simulink model "ESP_RTW"  (Simulink 10.1)
settings: Solver=ode1  StartTime=0.0  StopTime=inf  FixedStep=0.001  RelTol=1e-3
PreLoadFcn:
  | vehicle = 'Car'; if ~length(which('cmcmd')), cmenv; end
  | ESP_RTW_bus
  | ESP_RTW_params
InitFcn:
  | vehicle = 'Car'; if ~length(which('cmcmd')), cmenv; end
  | ESP_RTW_bus
  | ESP_RTW_params
values from neighbouring files (symbols this model uses):
  Area_Front = 23    [ESP_RTW_params.m]
  Area_Rear = 23    [ESP_RTW_params.m]
  ay_max_off = 4.0    (= 4)    [ESP_RTW_params.m]
  ay_max_on = 4.8    [ESP_RTW_params.m]
  ay_per_mu_max_off = 6    [ESP_RTW_params.m]
  ay_per_mu_max_on = 7    [ESP_RTW_params.m]
  Brake_ratio = 0.7    [ESP_RTW_params.m]
  brake_valve_ctrl_kP = 0.5    [ESP_RTW_params.m]
  cat1mode1_higher = 9    [ESP_RTW_params.m]
  cat1mode1_lower = 8    [ESP_RTW_params.m]
  cat1mode2_higher = 6    [ESP_RTW_params.m]
  cat1mode2_lower = 5    [ESP_RTW_params.m]
  cat1mode3_higher = 4    [ESP_RTW_params.m]
  cat1mode3_lower = 3    [ESP_RTW_params.m]
  cat2mode1_higher = 6    [ESP_RTW_params.m]
  cat2mode1_lower = 5.5    [ESP_RTW_params.m]
  cat2mode2_higher = 3    [ESP_RTW_params.m]
  cat2mode2_lower = 2.5    [ESP_RTW_params.m]
  cat2mode3_higher = 1    [ESP_RTW_params.m]
  cat2mode3_lower = 0.5    [ESP_RTW_params.m]
  delta_vel = 10    [ESP_RTW_params.m]
  diff_lock_fac = 1000    [ESP_RTW_params.m]
  diff_lock_off = 3    [ESP_RTW_params.m]
  diff_lock_on = 4    [ESP_RTW_params.m]
  ESP_ctrl_kD = 0    [ESP_RTW_params.m]
  ESP_ctrl_kI = -0.0001    [ESP_RTW_params.m]
  ESP_ctrl_kP = 0.4    [ESP_RTW_params.m]
  ESP_ctrl_restore_kI = 0.6    [ESP_RTW_params.m]
  ESP_min_throttle_fac = 0    [ESP_RTW_params.m]
  f_ax = 0.003    [ESP_RTW_params.m]
  f_slip = 1    [ESP_RTW_params.m]
  g = 9.81    [ESP_RTW_params.m]
  higherlimit_highvel = 2    [ESP_RTW_params.m]
  higherlimit_lowvel = 7    [ESP_RTW_params.m]
  highervel_fac = 0.04    [ESP_RTW_params.m]
  highervelocity_fac = 1.04    [ESP_RTW_params.m]
  limit_acc = 2    [ESP_RTW_params.m]
  limit_selectlow = 38    [ESP_RTW_params.m]
  limit_starting = 10    [ESP_RTW_params.m]
  limit_vdiff = 1    [ESP_RTW_params.m]
  locktime_throttle = 2    [ESP_RTW_params.m]
  lowerlimit_highvel = 1    [ESP_RTW_params.m]
  lowerlimit_lowvel = 6    [ESP_RTW_params.m]
  lowervel_fac = 0.02    [ESP_RTW_params.m]
  lowervelocity_fac = 1.02    [ESP_RTW_params.m]
  min_throttle = 0.05    [ESP_RTW_params.m]
  MPS2KMPH = 3.6    [ESP_RTW_params.m]
  MSR_ctrl_kD = 0    [ESP_RTW_params.m]
  MSR_ctrl_kI = 0    [ESP_RTW_params.m]
  MSR_ctrl_kP = 0.1    [ESP_RTW_params.m]
  MSR_min_throttle_fac = 0.2    [ESP_RTW_params.m]
  PID_kD_sideslip = 0    [ESP_RTW_params.m]
  PID_kD_yawrate = 0    [ESP_RTW_params.m]
  PID_kI_sideslip = 0    [ESP_RTW_params.m]
  PID_kI_yawrate = 0    [ESP_RTW_params.m]
  PID_kP_sideslip = 2550*0.55    (= 1402.5)    [ESP_RTW_params.m]
  PID_kP_yawrate = 6650*0.275    (= 1828.75)    [ESP_RTW_params.m]
  RADpS2RpM = 60/(2*pi)    (= 9.54929658551)    [ESP_RTW_params.m]
  rBrake = 0.1    [ESP_RTW_params.m]
  RpM2RADpS = (2*pi)/60    (= 0.10471975512)    [ESP_RTW_params.m]
  SH_SL_switch = 15    [ESP_RTW_params.m]
  sideslip_vel_corr = 5/6    (= 0.833333333333)    [ESP_RTW_params.m]
  sidesplip_deviation_max = 3    [ESP_RTW_params.m]
  sku_HA = 0.08   +offset    (= 0.08)    [ESP_RTW_params.m]
  sku_off_HA = 0.04   +offset    (= 0.04)    [ESP_RTW_params.m]
  sku_off_VA = 0.03   +offset    (= 0.03)    [ESP_RTW_params.m]
  sku_VA = 0.10   +offset    (= 0.1)    [ESP_RTW_params.m]
  SteerAng_Out = [-0.6 -0.6 -0.5 -0.41 -0.34 -0.27 -0.2 -0.13 -0.06 0 0.06 0.13 0.2 0.27 0.34 0.41 0.5 0.6 0.6]    [ESP_RTW_params.m]
  SteerWheelAng_In = [-15 -8 -7 -6 -5 -4 -3 -2 -1 0 1 2 3 4 5 6 7 8 15]    [ESP_RTW_params.m]
  t_Sensor = triggertime    (= 0.001)    [ESP_RTW_params.m]
  threshold_carpitch_off = 0.05    [ESP_RTW_params.m]
  threshold_carpitch_on = 0.1    [ESP_RTW_params.m]
  threshold_deceleration = -1    [ESP_RTW_params.m]
  threshold_eng_trq_off = 25    [ESP_RTW_params.m]
  threshold_eng_trq_on = 30    [ESP_RTW_params.m]
  threshold_velocity_off = -0.01    [ESP_RTW_params.m]
  threshold_velocity_on = 0.01    [ESP_RTW_params.m]
  v_min = 5    [ESP_RTW_params.m]
  Valve_LUTin_HA = [0 sku_off_HA-1e-5 ,sku_off_HA, sku_HA, sku_HA+1e-5, sko_HA-1e-5, sko_HA , sko_open_HA]    [ESP_RTW_params.m]
  Valve_LUTin_VA = [0 sku_off_VA-1e-5 ,sku_off_VA, sku_VA, sku_VA+1e-5, sko_VA-1e-5, sko_VA , sko_open_VA]    [ESP_RTW_params.m]
  ValveIn_abbau = 1    [ESP_RTW_params.m]
  ValveIn_aufbau_long = 0    [ESP_RTW_params.m]
  ValveIn_aufbau_short = 0.85    [ESP_RTW_params.m]
  ValveIn_LUTout_HA = [0, 0,   0.2,    0.6,    1.0,    1.0,     1.0,    1.0]    [ESP_RTW_params.m]
  ValveIn_LUTout_VA = [0, 0,   0.2,    0.4,    1.0,    1.0,     1.0,    1.0]    [ESP_RTW_params.m]
  ValveOut_abbau = 1    [ESP_RTW_params.m]
  ValveOut_aufbau_long = 0    [ESP_RTW_params.m]
  ValveOut_aufbau_short = 0.85    [ESP_RTW_params.m]
  ValveOut_LUTout_HA = [0, 0,   0,      0,      0,     0,      0.3,    1.0]    [ESP_RTW_params.m]
  ValveOut_LUTout_VA = [0, 0,   0,      0,      0,     0,      0.3,    1.0]    [ESP_RTW_params.m]
  vel_char_lim_high = 150    [ESP_RTW_params.m]
  vel_char_lim_low = 25    [ESP_RTW_params.m]
  wheelspeed_filter_denom = [1 1]    [ESP_RTW_params.m]
  wheelspeed_filter_num = [ones(1,20)/20]    [ESP_RTW_params.m]
  yawrate_deviation_max = 1    [ESP_RTW_params.m]
  yawrate_vel_corr = 0.5    [ESP_RTW_params.m]
undefined symbols (not defined in the file or in its folder): InitialConditionForIntegrator
libraries: CarMaker4SL x133, simulink x47, simulink_extras x6
(part 2 of 4)

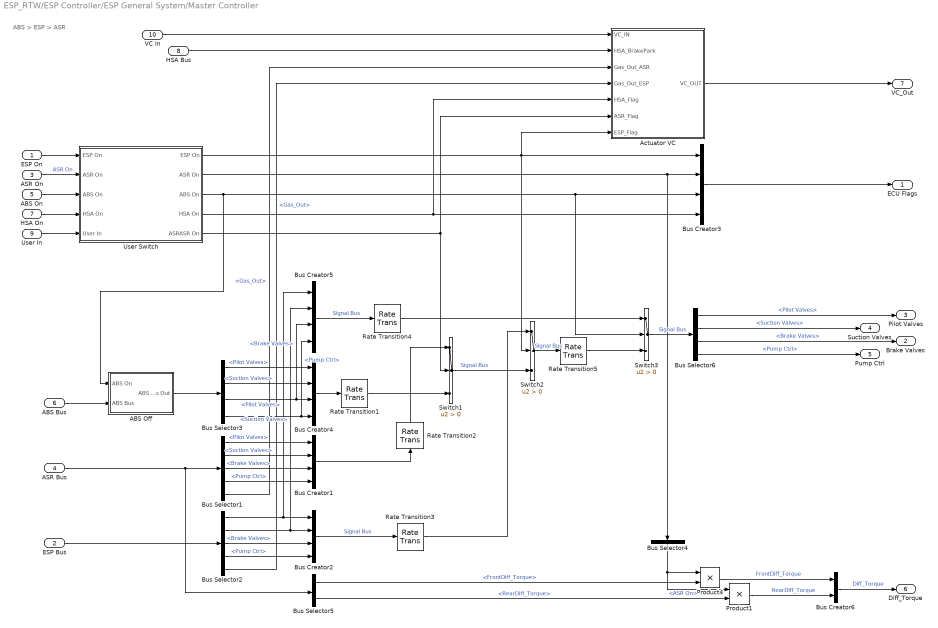
== system ESP_RTW/ESP Controller/ESP General System/Master Controller ==
  note: ABS > ESP > ASR
  ESP On : Inport
  ESP Bus : Inport  Port=2
  ASR On : Inport  Port=3
  ASR Bus : Inport  Port=4
  ABS On : Inport  Port=5
  ABS Bus : Inport  Port=6
  HSA On : Inport  Port=7
  HSA Bus : Inport  Port=8
  User In : Inport  Port=9
  VC In : Inport  Port=10
  ABS Off : Subsystem
  Actuator VC : Subsystem
  Bus Creator{1..5} (5 alike) : BusCreator  Inputs=4
  Bus Creator6 : BusCreator  Inputs=2
  Bus Selector1 : BusSelector  OutputSignals=Pilot Valves,Suction Valves,Brake Valves,Pump Ctrl,Gas_Out
  Bus Selector2 : BusSelector  OutputSignals=Pilot Valves,Suction Valves,Brake Valves,Pump Ctrl,Gas_Out
  Bus Selector3 : BusSelector  OutputSignals=Pilot Valves,Suction Valves,Brake Valves,Pump Ctrl
  Bus Selector4 : BusSelector  OutputSignals=ASR On
  Bus Selector5 : BusSelector  OutputSignals=Diff_Torque.FrontDiff_Torque,Diff_Torque.RearDiff_Torque
  Bus Selector6 : BusSelector  OutputSignals=Pilot Valves,Suction Valves,Brake Valves,Pump Ctrl
  Product1 : Product  RndMeth=Zero
  Product4 : Product  RndMeth=Zero
  Rate Transition{1..5} (5 alike) : RateTransition
  Switch1 : Switch  Criteria=u2 > Threshold
  Switch2 : Switch  Criteria=u2 > Threshold
  Switch3 : Switch  Criteria=u2 > Threshold
  User Switch : Subsystem
  ECU Flags : Outport  VectorParamsAs1DForOutWhenUnconnected=off
  Brake Valves : Outport  Port=2  VectorParamsAs1DForOutWhenUnconnected=off
  Pilot Valves : Outport  Port=3  VectorParamsAs1DForOutWhenUnconnected=off
  Suction Valves : Outport  Port=4  VectorParamsAs1DForOutWhenUnconnected=off
  Pump Ctrl : Outport  Port=5  VectorParamsAs1DForOutWhenUnconnected=off
  Diff_Torque : Outport  Port=6  VectorParamsAs1DForOutWhenUnconnected=off
  VC_Out : Outport  Port=7  VectorParamsAs1DForOutWhenUnconnected=off
  wires:
  Rate Transition5/1 -> Switch3/3
  Rate Transition4/1 -> Switch3/1
  Rate Transition3/1 -> Switch2/1
  ABS Off/1(ABS Bus Out) -> Bus Selector3/1
  Bus Selector4/1 -> Product4/1, Product1/1  "<ASR On>"
  Bus Creator6/1 -> Diff_Torque/1  "Diff_Torque"
  Product1/1 -> Bus Creator6/2  "RearDiff_Torque"
  Product4/1 -> Bus Creator6/1  "FrontDiff_Torque"
  Bus Selector5/2 -> Product1/2  "<RearDiff_Torque>"
  Bus Selector5/1 -> Product4/2  "<FrontDiff_Torque>"
  User Switch/4("HSA On ") -> Actuator VC/5(HSA_Flag), Bus Creator3/4
  HSA On/1 -> User Switch/4(HSA On)
  HSA Bus/1 -> Actuator VC/2(HSA_BrakePark)
  User Switch/2("ASR On ") -> Bus Selector4/1, Bus Creator3/2
  User In/1 -> User Switch/5(User In)
  ABS On/1 -> User Switch/3(ABS On)
  ASR On/1 -> User Switch/2(ASR On)  "ASR On"
  ESP On/1 -> User Switch/1(ESP On)
  User Switch/1("ESP On ") -> Switch2/2, Bus Creator3/1, Actuator VC/7(ESP_Flag)
  User Switch/5(ASRASR On) -> Switch1/2, Actuator VC/6(ASR_Flag)
  User Switch/3("ABS On ") -> Switch3/2, Bus Creator3/3, ABS Off/1(ABS On)
  Bus Selector2/5 -> Actuator VC/4(Gas_Out_ESP)  "<Gas_Out>"
  Bus Selector1/5 -> Actuator VC/3(Gas_Out_ASR)  "<Gas_Out>"
  Switch3/1 -> Bus Selector6/1  "Signal Bus"
  Rate Transition1/1 -> Switch1/3
  Rate Transition2/1 -> Switch1/1
  Bus Creator4/1 -> Rate Transition1/1
  Bus Creator1/1 -> Rate Transition2/1
  Bus Creator5/1 -> Rate Transition4/1  "Signal Bus"
  Switch2/1 -> Rate Transition5/1  "Signal Bus"
  Bus Selector1/4 -> Bus Creator1/4  "<Pump Ctrl>"
  Bus Selector1/3 -> Bus Creator1/3  "<Brake Valves>"
  Bus Selector1/2 -> Bus Creator1/2  "<Suction Valves>"
  Bus Selector1/1 -> Bus Creator1/1  "<Pilot Valves>"
  ASR Bus/1 -> Bus Selector1/1, Bus Selector5/1
  Bus Creator2/1 -> Rate Transition3/1  "Signal Bus"
  Switch1/1 -> Switch2/3  "Signal Bus"
  Bus Selector3/2 -> Bus Creator4/2  "<Suction Valves>"
  Bus Selector3/1 -> Bus Creator4/1  "<Pilot Valves>"
  ABS Bus/1 -> ABS Off/2(ABS Bus)
  Bus Selector3/4 -> Bus Creator4/4, Bus Creator5/4  "<Pump Ctrl>"
  Bus Selector3/3 -> Bus Creator4/3, Bus Creator5/3  "<Brake Valves>"
  Bus Selector6/4 -> Pump Ctrl/1  "<Pump Ctrl>"
  Bus Selector6/3 -> Brake Valves/1  "<Brake Valves>"
  Bus Selector6/2 -> Suction Valves/1  "<Suction Valves>"
  Bus Selector6/1 -> Pilot Valves/1  "<Pilot Valves>"
  Bus Selector2/4 -> Bus Creator2/4  "<Pump Ctrl>"
  Bus Selector2/3 -> Bus Creator2/3  "<Brake Valves>"
  Bus Selector2/2 -> Bus Creator2/2, Bus Creator5/2  "<Suction Valves>"
  Bus Selector2/1 -> Bus Creator2/1, Bus Creator5/1  "<Pilot Valves>"
  ESP Bus/1 -> Bus Selector2/1
  VC In/1 -> Actuator VC/1(VC_IN)
  Actuator VC/1(VC_OUT) -> VC_Out/1
  Bus Creator3/1 -> ECU Flags/1

== system ESP_RTW/ESP Controller/ESP General System/Signal Handling ==
  ESP In : Inport
  Vehicle Params : Inport  Port=2
  " " : simulink_extras/Transformations/Degrees to Radians
  "  " : simulink_extras/Transformations/Degrees to Radians
  "   " : Gain  Gain=RpM2RADpS
  "     " : Gain  Gain=RpM2RADpS
  "      " : Gain  Gain=RpM2RADpS
  Bus Creator : BusCreator  Inputs=4
  Bus Creator1 : BusCreator  Inputs=4
  Bus Creator2 : BusCreator  Inputs=6
  Bus Creator3 : BusCreator  Inputs=2
  Bus Creator4 : BusCreator  Inputs=2
  Bus Creator5 : BusCreator  Inputs=1
  Bus Selector1 : BusSelector  OutputSignals=WheelSpd FL [rpm],WheelSpd FR [rpm],WheelSpd RL [rpm],WheelSpd RR [rpm],Master Cylinder Pressure [bar],Throttle Valve Position [%],Sensor Longitudinal acceleration [g],Engine Speed [rpm],GearState [-],Torque Converter Speed [rpm],Sensor YawRate [degs],Steering Wheel Angle [deg],Sensor Lateral acceleration [g],Cylinder Pressure FL [bar],Cylinder Pressure FR [bar],Cylinder Pressure RL [bar],Cylinder Pressure RR [bar],Engine crankshaft output torque [Nm]
  Bus Selector2 : BusSelector  OutputSignals=SteeringGeometry
  Bus Selector3 : BusSelector  OutputSignals=SteerWheelAng_In,SteerAng_Out
  Gain2 : Gain  Gain=g  SaturateOnIntegerOverflow=on  OutDataTypeStr=Inherit: Same as input  ParamDataTypeStr=Inherit: Same as input
  Gain7 : Gain  Gain=g  SaturateOnIntegerOverflow=on  OutDataTypeStr=Inherit: Same as input  ParamDataTypeStr=Inherit: Same as input
  Lookup Table Dynamic : simulink/Lookup Tables/Lookup Table Dynamic  LookUpMeth=Interpolation-Use End Values  OutDataTypeStr=fixdt('double')  OutputDataTypeScalingMode=Specify via dialog  OutDataType=fixdt('double')  OutScaling=2^-10  DoSatur=off
  Termiator : Terminator
  Terminator1 : Terminator
  Terminator2 : Terminator
  Terminator4 : Terminator
  rpmin2rad/s : Gain  Gain=RpM2RADpS
  vquer_VA3 : Gain  Gain=0.01
  Signal Bus ESP : Outport  VectorParamsAs1DForOutWhenUnconnected=off
  Signal Bus ASR : Outport  Port=2  VectorParamsAs1DForOutWhenUnconnected=off
  Signal Bus ABS : Outport  Port=3  VectorParamsAs1DForOutWhenUnconnected=off
  Signal Bus HSA : Outport  Port=4  VectorParamsAs1DForOutWhenUnconnected=off
  wires:
  Bus Selector3/1 -> Lookup Table Dynamic/2  "<SteerWheelAng_In>"
  Bus Selector3/2 -> Lookup Table Dynamic/3  "<SteerAng_Out>"
  Bus Selector2/1 -> Bus Selector3/1  "<SteeringGeometry>"
  Vehicle Params/1 -> Bus Selector2/1
  Bus Creator5/1 -> Signal Bus HSA/1
  Bus Creator4/1 -> Signal Bus ABS/1
  Bus Selector1/18 -> Bus Creator5/1  "<Engine crankshaft output torque [Nm]>"
  Bus Creator3/1 -> Signal Bus ASR/1
  Bus Creator/1 -> Bus Creator3/1, Bus Creator4/1  "WheelSpeeds"
  Bus Creator2/1 -> Signal Bus ESP/1
  Bus Creator1/1 -> Bus Creator2/6  "Wheel Cylinder Pressure"
  Bus Selector1/14 -> Bus Creator1/1  "<Cylinder Pressure FL [bar]>"
  Bus Selector1/16 -> Bus Creator1/3  "<Cylinder Pressure RL [bar]>"
  Bus Selector1/17 -> Bus Creator1/4  "<Cylinder Pressure RR [bar]>"
  Bus Selector1/15 -> Bus Creator1/2  "<Cylinder Pressure FR [bar]>"
  vquer_VA3/1 -> Bus Creator3/2, Bus Creator2/1  "Throttle Position"
  Gain2/1 -> Bus Creator2/4  "ay [m/s^2]"
  " "/1 -> Bus Creator2/2  "Yaw Rate"
  Lookup Table Dynamic/1 -> Bus Creator2/3  "Steer Angle"
  ESP In/1 -> Bus Selector1/1
  Bus Selector1/6 -> vquer_VA3/1  "<Throttle Valve Position [%]>"
  Gain7/1 -> Bus Creator2/5, Bus Creator4/2  "ax [m/s^2]"
  "      "/1 -> Bus Creator/4  "WheelSpd_RR"
  "     "/1 -> Bus Creator/3  "WheelSpd_RL"
  "   "/1 -> Bus Creator/2  "WheelSpd_FR"
  Bus Selector1/13 -> Gain2/1  "<Sensor Lateral acceleration [g]>"
  Bus Selector1/12 -> "  "/1  "<Steering Wheel Angle [deg]>"
  Bus Selector1/11 -> " "/1  "<Sensor YawRate [degs]>"
  Bus Selector1/10 -> Termiator/1  "<Torque Converter Speed [rpm]>"
  Bus Selector1/9 -> Terminator1/1  "<GearState [-]>"
  Bus Selector1/8 -> Terminator2/1  "<Engine Speed [rpm]>"
  Bus Selector1/5 -> Terminator4/1  "<Master Cylinder Pressure [bar]>"
  Bus Selector1/7 -> Gain7/1  "<Sensor Longitudinal acceleration [g]>"
  Bus Selector1/4 -> "      "/1  "<WheelSpd RR [rpm]>"
  Bus Selector1/3 -> "     "/1  "<WheelSpd RL [rpm]>"
  Bus Selector1/2 -> "   "/1  "<WheelSpd FR [rpm]>"
  Bus Selector1/1 -> rpmin2rad/s/1  "<WheelSpd FL [rpm]>"
  rpmin2rad/s/1 -> Bus Creator/1  "WheelSpd_FL"
  "  "/1 -> Lookup Table Dynamic/1

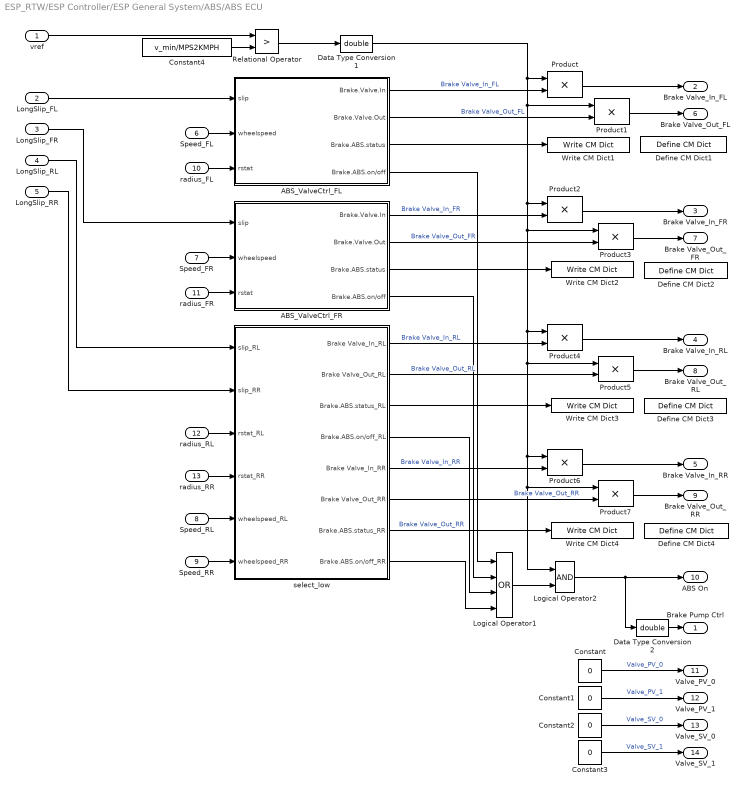
== system ESP_RTW/ESP Controller/ESP General System/ABS/ABS ECU ==
  vref : Inport
  LongSlip_FL : Inport  Port=2
  LongSlip_FR : Inport  Port=3
  LongSlip_RL : Inport  Port=4
  LongSlip_RR : Inport  Port=5
  Speed_FL : Inport  Port=6
  Speed_FR : Inport  Port=7
  Speed_RL : Inport  Port=8
  Speed_RR : Inport  Port=9
  radius_FL : Inport  Port=10
  radius_FR : Inport  Port=11
  radius_RL : Inport  Port=12
  radius_RR : Inport  Port=13
  ABS_ValveCtrl_FL : Subsystem
  ABS_ValveCtrl_FR : Subsystem
  Constant{,1..3} (4 alike) : Constant  Value=0
  Constant4 : Constant  Value=v_min/MPS2KMPH
  Data Type Conversion1 : DataTypeConversion  OutDataTypeStr=double
  Data Type Conversion2 : DataTypeConversion  OutDataTypeStr=double
  Define CM Dict1 : CarMaker4SL/Define CM Dict  xname=ESP.ABS.Status_FL  xmono=off  xtype=Char  xdvaplace=None  xnstates=4  xfirststate=0  xinitial=0
  Define CM Dict2 : CarMaker4SL/Define CM Dict  xname=ESP.ABS.Status_FR  xmono=off  xtype=Char  xdvaplace=None  xnstates=4  xfirststate=0  xinitial=0
  Define CM Dict3 : CarMaker4SL/Define CM Dict  xname=ESP.ABS.Status_RL  xmono=off  xtype=Char  xdvaplace=None  xnstates=4  xfirststate=0  xinitial=0
  Define CM Dict4 : CarMaker4SL/Define CM Dict  xname=ESP.ABS.Status_RR  xmono=off  xtype=Char  xdvaplace=None  xnstates=4  xfirststate=0  xinitial=0
  Logical Operator1 : Logic  Operator=OR  Inputs=4  AllPortsSameDT=off
  Logical Operator2 : Logic  AllPortsSameDT=off
  Product{,1..7} (8 alike) : Product  SaturateOnIntegerOverflow=on  OutDataTypeStr=Inherit: Same as first input
  Relational Operator : RelationalOperator  Operator=>  RndMeth=Nearest
  Write CM Dict1 : CarMaker4SL/Write CM Dict  xname=ESP.ABS.Status_FL  xsync=off
  Write CM Dict2 : CarMaker4SL/Write CM Dict  xname=ESP.ABS.Status_FR  xsync=off
  Write CM Dict3 : CarMaker4SL/Write CM Dict  xname=ESP.ABS.Status_RL  xsync=off
  Write CM Dict4 : CarMaker4SL/Write CM Dict  xname=ESP.ABS.Status_RR  xsync=off
  select_low : Subsystem
  Brake Pump Ctrl : Outport  VectorParamsAs1DForOutWhenUnconnected=off
  Brake Valve_In_FL : Outport  Port=2  VectorParamsAs1DForOutWhenUnconnected=off
  Brake Valve_In_FR : Outport  Port=3  VectorParamsAs1DForOutWhenUnconnected=off
  Brake Valve_In_RL : Outport  Port=4  VectorParamsAs1DForOutWhenUnconnected=off
  Brake Valve_In_RR : Outport  Port=5  VectorParamsAs1DForOutWhenUnconnected=off
  Brake Valve_Out_FL : Outport  Port=6  VectorParamsAs1DForOutWhenUnconnected=off
  Brake Valve_Out_FR : Outport  Port=7  VectorParamsAs1DForOutWhenUnconnected=off
  Brake Valve_Out_RL : Outport  Port=8  VectorParamsAs1DForOutWhenUnconnected=off
  Brake Valve_Out_RR : Outport  Port=9  VectorParamsAs1DForOutWhenUnconnected=off
  ABS On : Outport  Port=10  VectorParamsAs1DForOutWhenUnconnected=off
  Valve_PV_0 : Outport  Port=11  VectorParamsAs1DForOutWhenUnconnected=off
  Valve_PV_1 : Outport  Port=12  VectorParamsAs1DForOutWhenUnconnected=off
  Valve_SV_0 : Outport  Port=13  VectorParamsAs1DForOutWhenUnconnected=off
  Valve_SV_1 : Outport  Port=14  VectorParamsAs1DForOutWhenUnconnected=off
  wires:
  Logical Operator2/1 -> Data Type Conversion2/1, ABS On/1
  Logical Operator1/1 -> Logical Operator2/2
  Constant3/1 -> Valve_SV_1/1  "Valve_SV_1"
  Constant2/1 -> Valve_SV_0/1  "Valve_SV_0"
  Constant1/1 -> Valve_PV_1/1  "Valve_PV_1"
  Constant/1 -> Valve_PV_0/1  "Valve_PV_0"
  vref/1 -> Relational Operator/1
  Speed_RR/1 -> select_low/6(wheelspeed_RR)
  Speed_RL/1 -> select_low/5(wheelspeed_RL)
  radius_RR/1 -> select_low/4(rstat_RR)
  radius_RL/1 -> select_low/3(rstat_RL)
  radius_FR/1 -> ABS_ValveCtrl_FR/3(rstat)
  Speed_FR/1 -> ABS_ValveCtrl_FR/2(wheelspeed)
  radius_FL/1 -> ABS_ValveCtrl_FL/3(rstat)
  Speed_FL/1 -> ABS_ValveCtrl_FL/2(wheelspeed)
  Product2/1 -> Brake Valve_In_FR/1
  Product/1 -> Brake Valve_In_FL/1
  ABS_ValveCtrl_FL/3(Brake.ABS.status) -> Write CM Dict1/1
  LongSlip_RR/1 -> select_low/2(slip_RR)
  LongSlip_RL/1 -> select_low/1(slip_RL)
  LongSlip_FR/1 -> ABS_ValveCtrl_FR/1(slip)
  LongSlip_FL/1 -> ABS_ValveCtrl_FL/1(slip)
  Product1/1 -> Brake Valve_Out_FL/1
  Product3/1 -> Brake Valve_Out_FR/1
  Product4/1 -> Brake Valve_In_RL/1
  Product5/1 -> Brake Valve_Out_RL/1
  Product6/1 -> Brake Valve_In_RR/1
  Product7/1 -> Brake Valve_Out_RR/1
  select_low/6(Brake Valve_Out_RR) -> Product7/2  "Brake Valve_Out_RR"
  select_low/5(Brake Valve_In_RR) -> Product6/2  "Brake Valve_In_RR"
  select_low/2(Brake Valve_Out_RL) -> Product5/2  "Brake Valve_Out_RL"
  select_low/1(Brake Valve_In_RL) -> Product4/2  "Brake Valve_In_RL"
  ABS_ValveCtrl_FR/2(Brake.Valve.Out) -> Product3/2  "Brake Valve_Out_FR"
  ABS_ValveCtrl_FR/1(Brake.Valve.In) -> Product2/2  "Brake Valve_In_FR"
  ABS_ValveCtrl_FL/2(Brake.Valve.Out) -> Product1/2  "Brake Valve_Out_FL"
  ABS_ValveCtrl_FL/1(Brake.Valve.In) -> Product/2  "Brake Valve_In_FL"
  Relational Operator/1 -> Data Type Conversion1/1
  Constant4/1 -> Relational Operator/2
  select_low/8(Brake.ABS.on/off_RR) -> Logical Operator1/4
  select_low/4(Brake.ABS.on/off_RL) -> Logical Operator1/3
  ABS_ValveCtrl_FR/4(Brake.ABS.on/off) -> Logical Operator1/2
  ABS_ValveCtrl_FL/4(Brake.ABS.on/off) -> Logical Operator1/1
  ABS_ValveCtrl_FR/3(Brake.ABS.status) -> Write CM Dict2/1
  select_low/3(Brake.ABS.status_RL) -> Write CM Dict3/1
  select_low/7(Brake.ABS.status_RR) -> Write CM Dict4/1  "Brake Valve_Out_RR"
  Data Type Conversion1/1 -> Product1/1, Product2/1, Product3/1, Product4/1, Product5/1, Logical Operator2/1, Product7/1, Product6/1, Product/1
  Data Type Conversion2/1 -> Brake Pump Ctrl/1

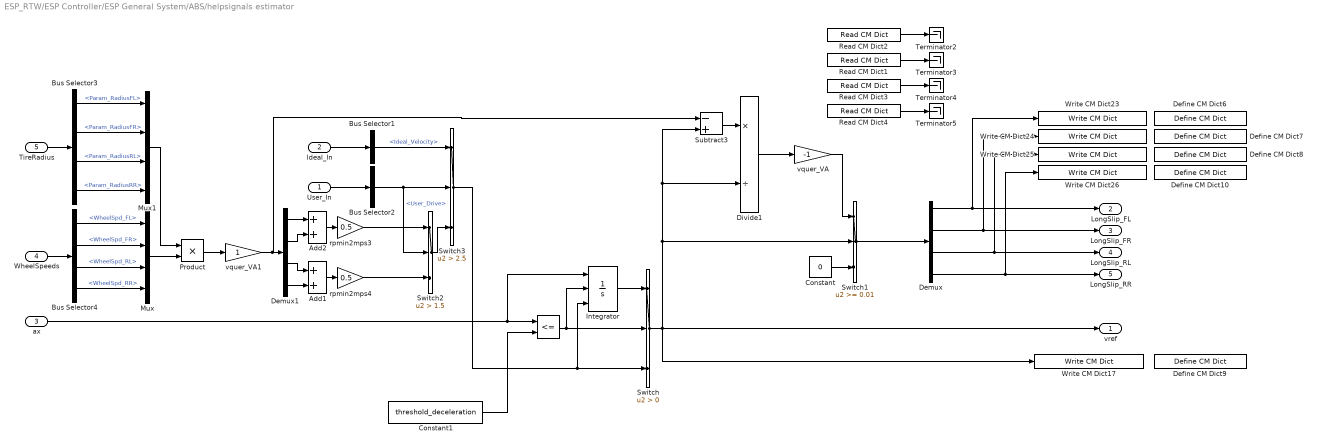
== system ESP_RTW/ESP Controller/ESP General System/ABS/helpsignals estimator ==
  User_In : Inport
  Ideal_In : Inport  Port=2
  ax : Inport  Port=3
  WheelSpeeds : Inport  Port=4
  TireRadius : Inport  Port=5
  " " : RelationalOperator  Operator=<=  OutDataTypeStr=boolean  RndMeth=Nearest
  Add1 : Sum
  Add2 : Sum
  Bus Selector1 : BusSelector  OutputSignals=Ideal_Velocity.Ideal_Velocity
  Bus Selector2 : BusSelector  OutputSignals=User_Drive
  Bus Selector3 : BusSelector  OutputSignals=Param_RadiusFL,Param_RadiusFR,Param_RadiusRL,Param_RadiusRR
  Bus Selector4 : BusSelector  OutputSignals=WheelSpd_FL,WheelSpd_FR,WheelSpd_RL,WheelSpd_RR
  Constant : Constant  Value=0
  Constant1 : Constant  Value=threshold_deceleration
  Define CM Dict10 : CarMaker4SL/Define CM Dict  xname=ESP.ABS.LongSlip_RR  xmono=off  xtype=Double4  xdvaplace=VC  xnstates=0  xfirststate=0  xinitial=0
  Define CM Dict6 : CarMaker4SL/Define CM Dict  xname=ESP.ABS.LongSlip_FL  xmono=off  xtype=Double4  xdvaplace=VC  xnstates=0  xfirststate=0  xinitial=0
  Define CM Dict7 : CarMaker4SL/Define CM Dict  xname=ESP.ABS.LongSlip_FR  xmono=off  xtype=Double4  xdvaplace=VC  xnstates=0  xfirststate=0  xinitial=0
  Define CM Dict8 : CarMaker4SL/Define CM Dict  xname=ESP.ABS.LongSlip_RL  xmono=off  xtype=Double4  xdvaplace=VC  xnstates=0  xfirststate=0  xinitial=0
  Define CM Dict9 : CarMaker4SL/Define CM Dict  xname=ESP.ABS.v_ref  xunit=m/s  xmono=off  xtype=Double4  xdvaplace=VC  xnstates=0  xfirststate=0  xinitial=0
  Demux : Demux
  Demux1 : Demux
  Divide1 : Product  Inputs=*/
  Integrator : Integrator  ExternalReset=rising  InitialConditionSource=external
  Mux : Mux
  Mux1 : Mux
  Product : Product  RndMeth=Zero
  Read CM Dict1 : CarMaker4SL/Read CM Dict  xname=Car.LongSlipFR  xsync=off
  Read CM Dict2 : CarMaker4SL/Read CM Dict  xname=Car.LongSlipFL  xsync=off
  Read CM Dict3 : CarMaker4SL/Read CM Dict  xname=Car.LongSlipRL  xsync=off
  Read CM Dict4 : CarMaker4SL/Read CM Dict  xname=Car.LongSlipRR  xsync=off
  Subtract3 : Sum  Inputs=-+
  Switch : Switch  Criteria=u2 > Threshold
  Switch1 : Switch  Threshold=0.01
  Switch2 : Switch  Criteria=u2 > Threshold  Threshold=1.5
  Switch3 : Switch  Criteria=u2 > Threshold  Threshold=2.5
  Terminator{2..5} (4 alike) : Terminator
  Write CM Dict17 : CarMaker4SL/Write CM Dict  xname=ESP.ABS.v_ref  xsync=off
  Write CM Dict23 : CarMaker4SL/Write CM Dict  xname=ESP.ABS.LongSlip_FL  xsync=off
  Write CM Dict24 : CarMaker4SL/Write CM Dict  xname=ESP.ABS.LongSlip_FR  xsync=off
  Write CM Dict25 : CarMaker4SL/Write CM Dict  xname=ESP.ABS.LongSlip_RL  xsync=off
  Write CM Dict26 : CarMaker4SL/Write CM Dict  xname=ESP.ABS.LongSlip_RR  xsync=off
  rpmin2mps3 : Gain  Gain=0.5
  rpmin2mps4 : Gain  Gain=0.5
  vquer_VA : Gain  Gain=-1
  vquer_VA1 : Gain
  vref : Outport  VectorParamsAs1DForOutWhenUnconnected=off
  LongSlip_FL : Outport  Port=2  VectorParamsAs1DForOutWhenUnconnected=off
  LongSlip_FR : Outport  Port=3  VectorParamsAs1DForOutWhenUnconnected=off
  LongSlip_RL : Outport  Port=4  VectorParamsAs1DForOutWhenUnconnected=off
  LongSlip_RR : Outport  Port=5  VectorParamsAs1DForOutWhenUnconnected=off
  wires:
  Integrator/1 -> Switch/1
  Constant1/1 -> " "/2
  rpmin2mps4/1 -> Switch2/3
  rpmin2mps3/1 -> Switch2/1
  Bus Selector4/1 -> Mux/1  "<WheelSpd_FL>"
  Bus Selector4/2 -> Mux/2  "<WheelSpd_FR>"
  Bus Selector4/3 -> Mux/3  "<WheelSpd_RL>"
  Bus Selector4/4 -> Mux/4  "<WheelSpd_RR>"
  WheelSpeeds/1 -> Bus Selector4/1
  Bus Selector3/1 -> Mux1/1  "<Param_RadiusFL>"
  Bus Selector3/4 -> Mux1/4  "<Param_RadiusRR>"
  Bus Selector3/3 -> Mux1/3  "<Param_RadiusRL>"
  Bus Selector3/2 -> Mux1/2  "<Param_RadiusFR>"
  TireRadius/1 -> Bus Selector3/1
  Ideal_In/1 -> Bus Selector1/1
  Bus Selector1/1 -> Switch3/1  "<Ideal_Velocity>"
  Switch2/1 -> Switch3/3
  Add2/1 -> rpmin2mps3/1
  Bus Selector2/1 -> Switch3/2, Switch2/2  "<User_Drive>"
  Add1/1 -> rpmin2mps4/1
  User_In/1 -> Bus Selector2/1
  Demux1/2 -> Add2/2
  Demux1/1 -> Add2/1
  Read CM Dict4/1 -> Terminator5/1
  Read CM Dict3/1 -> Terminator4/1
  Read CM Dict1/1 -> Terminator3/1
  Read CM Dict2/1 -> Terminator2/1
  " "/1 -> Switch/2, Integrator/2
  vquer_VA1/1 -> Demux1/1, Subtract3/1
  Demux/4 -> Write CM Dict26/1, LongSlip_RR/1
  Demux/3 -> Write CM Dict25/1, LongSlip_RL/1
  Demux/2 -> Write CM Dict24/1, LongSlip_FR/1
  Demux/1 -> Write CM Dict23/1, LongSlip_FL/1
  Constant/1 -> Switch1/3
  Switch1/1 -> Demux/1
  Switch/1 -> Write CM Dict17/1, vref/1, Switch1/2, Divide1/2, Subtract3/2
  Demux1/4 -> Add1/2
  Demux1/3 -> Add1/1
  Switch3/1 -> Switch/3, Integrator/3
  ax/1 -> " "/1, Integrator/1
  vquer_VA/1 -> Switch1/1
  Divide1/1 -> vquer_VA/1
  Subtract3/1 -> Divide1/1
  Mux/1 -> Product/2
  Mux1/1 -> Product/1
  Product/1 -> vquer_VA1/1

== system ESP_RTW/ESP Controller/ESP General System/ASR/BMR ECU ==
  Throttle : Inport
  WheelVelocity [kmph] : Inport  Port=2
  User_In : Inport  Port=3
  Ideal_In : Inport  Port=4
  BMR Controller : Subsystem
  BMR logic : Subsystem
  Bus Creator : BusCreator  Inputs=8
  Bus Creator1 : BusCreator  Inputs=2
  Bus Creator2 : BusCreator  Inputs=2
  Bus Creator3 : BusCreator  Inputs=2
  Differential Lock : Subsystem
  Signal Mapping : Subsystem
  BMR On : Outport  VectorParamsAs1DForOutWhenUnconnected=off
  Brake Valves : Outport  Port=2  VectorParamsAs1DForOutWhenUnconnected=off
  Pilot Valves : Outport  Port=3  VectorParamsAs1DForOutWhenUnconnected=off
  Suctions Valves : Outport  Port=4  VectorParamsAs1DForOutWhenUnconnected=off
  Pump Ctrl : Outport  Port=5  VectorParamsAs1DForOutWhenUnconnected=off
  Diff_Torque : Outport  Port=6  VectorParamsAs1DForOutWhenUnconnected=off
  wires:
  User_In/1 -> Signal Mapping/1(User_In), Differential Lock/1(User_In), BMR Controller/1(User_In)
  BMR logic/2(BMR On) -> BMR On/1, BMR Controller/3(BMR On)
  BMR logic/1(mode) -> BMR Controller/2(mode)
  Throttle/1 -> BMR logic/5(Throttle position)
  Signal Mapping/4(v_UndrivenR) -> BMR logic/4(v_undrivenR)
  Signal Mapping/3(v_UndrivenL) -> BMR logic/3(v_undrivenL)
  Signal Mapping/2(v_DrivenR) -> BMR logic/2(v_drivenR), Differential Lock/3(v_DrivenR)
  Signal Mapping/1(v_DrivenL) -> BMR logic/1(v_drivenL), Differential Lock/2(v_DrivenL)
  Ideal_In/1 -> Signal Mapping/3(Ideal_In)
  Bus Creator3/1 -> Diff_Torque/1
  Differential Lock/2(RearDiff_Torque) -> Bus Creator3/2  "RearDiff_Torque"
  Differential Lock/1(FrontDiff_Torque) -> Bus Creator3/1  "FrontDiff_Torque"
  WheelVelocity [kmph]/1 -> Signal Mapping/2(WheelVelocity)
  Bus Creator1/1 -> Suctions Valves/1
  Bus Creator2/1 -> Pilot Valves/1
  BMR Controller/13(Pump Ctrl) -> Pump Ctrl/1  "PumpCtrl"
  BMR Controller/12(Valve_SV_1) -> Bus Creator1/2  "Valve_SV_1"
  BMR Controller/11(Valve_SV_0) -> Bus Creator1/1  "Valve_SV_0"
  BMR Controller/10(Valve_PV_1) -> Bus Creator2/2  "Valve_PV_1"
  BMR Controller/9(Valve_PV_0) -> Bus Creator2/1  "Valve_PV_0"
  BMR Controller/8(Brake Valve_Out_RR) -> Bus Creator/8  "Valve_Out_RR"
  BMR Controller/7(Brake Valve_Out_RL) -> Bus Creator/7  "Valve_Out_RL"
  BMR Controller/6(Brake Valve_Out_FR) -> Bus Creator/6  "Valve_Out_FR"
  BMR Controller/5(Brake Valve_Out_FL) -> Bus Creator/5  "Valve_Out_FL"
  BMR Controller/4(Brake Valve_In_RR) -> Bus Creator/4  "Valve_In_RR"
  BMR Controller/3(Brake Valve_In_RL) -> Bus Creator/3  "Valve_In_RL"
  BMR Controller/2(Brake Valve_In_FR) -> Bus Creator/2  "Valve_In_FR"
  BMR Controller/1(Brake Valve_In_FL) -> Bus Creator/1  "Valve_In_FL"
  Bus Creator/1 -> Brake Valves/1

== system ESP_RTW/ESP Controller/ESP General System/ASR/MSR ECU ==
  Throttle Position : Inport
  WheelVelocity [kmph] : Inport  Port=2
  User_In : Inport  Port=3
  Ideal_In : Inport  Port=4
  MSR logic : Subsystem
  MSR/Gas Controller : Subsystem
  Signal Mapping : Subsystem
  Gas_out : Outport  VectorParamsAs1DForOutWhenUnconnected=off
  MSR On : Outport  Port=2  VectorParamsAs1DForOutWhenUnconnected=off
  wires:
  MSR logic/3(hold torque) -> MSR/Gas Controller/4(hold Gas)
  MSR logic/2(reduce torque) -> MSR/Gas Controller/3(close Gas)
  MSR logic/1(Pseudo_slip) -> MSR/Gas Controller/2(Pseudo_Slip)
  Signal Mapping/4(v_UndrivenR) -> MSR logic/4(v_undrivenR)
  Signal Mapping/3(v_UndrivenL) -> MSR logic/3(v_undrivenL)
  Signal Mapping/2(v_DrivenR) -> MSR logic/2(v_drivenR)
  Signal Mapping/1(v_DrivenL) -> MSR logic/1(v_drivenL)
  Ideal_In/1 -> Signal Mapping/3(Ideal_In)
  User_In/1 -> Signal Mapping/2(User_In)
  WheelVelocity [kmph]/1 -> Signal Mapping/1(WheelVelocity)
  MSR/Gas Controller/2(Gas_Out) -> Gas_out/1
  MSR/Gas Controller/1(MSR_On) -> MSR On/1
  Throttle Position/1 -> MSR/Gas Controller/1(Throttle_position)

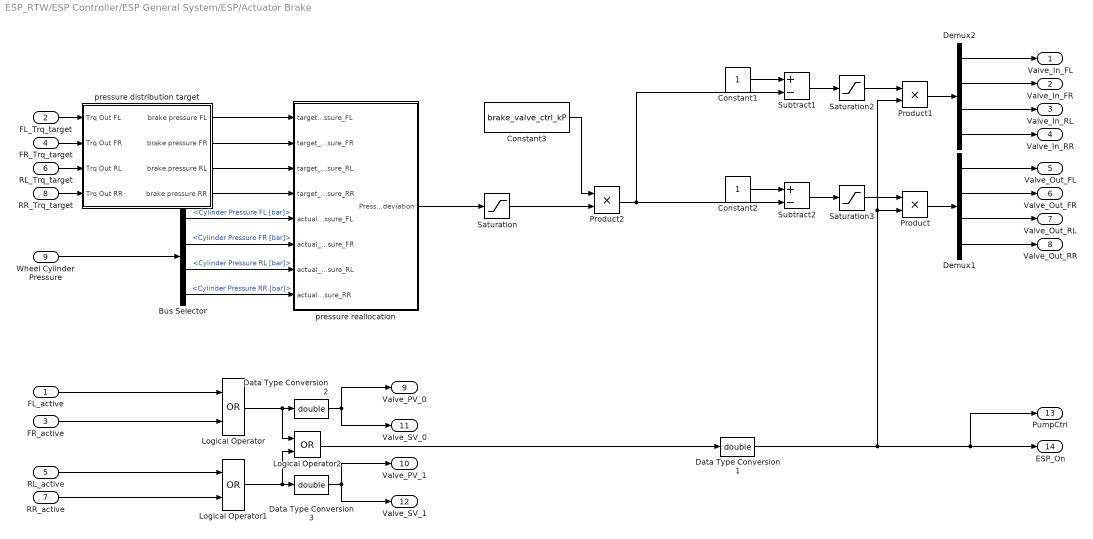
== system ESP_RTW/ESP Controller/ESP General System/ESP/Actuator Brake ==
  FL_active : Inport
  FL_Trq_target : Inport  Port=2
  FR_active : Inport  Port=3
  FR_Trq_target : Inport  Port=4
  RL_active : Inport  Port=5
  RL_Trq_target : Inport  Port=6
  RR_active : Inport  Port=7
  RR_Trq_target : Inport  Port=8
  Wheel Cylinder Pressure : Inport  Port=9
  Bus Selector : BusSelector  OutputSignals=Cylinder Pressure FL [bar],Cylinder Pressure FR [bar],Cylinder Pressure RL [bar],Cylinder Pressure RR [bar]
  Constant1 : Constant
  Constant2 : Constant
  Constant3 : Constant  Value=brake_valve_ctrl_kP
  Data Type Conversion1 : DataTypeConversion  OutDataTypeStr=double
  Data Type Conversion2 : DataTypeConversion  OutDataTypeStr=double
  Data Type Conversion3 : DataTypeConversion  OutDataTypeStr=double
  Demux1 : Demux
  Demux2 : Demux
  Logical Operator : Logic  Operator=OR  AllPortsSameDT=off
  Logical Operator1 : Logic  Operator=OR  AllPortsSameDT=off
  Logical Operator2 : Logic  Operator=OR  AllPortsSameDT=off
  Product : Product  RndMeth=Zero
  Product1 : Product  RndMeth=Zero
  Product2 : Product  RndMeth=Zero
  Saturation : Saturate  UpperLimit=500  LowerLimit=0
  Saturation2 : Saturate  UpperLimit=1  LowerLimit=0
  Saturation3 : Saturate  UpperLimit=1  LowerLimit=0
  Subtract1 : Sum  Inputs=+-
  Subtract2 : Sum  Inputs=+-
  pressure distribution target : Subsystem
  pressure reallocation : Subsystem
  Valve_In_FL : Outport  VectorParamsAs1DForOutWhenUnconnected=off
  Valve_In_FR : Outport  Port=2  VectorParamsAs1DForOutWhenUnconnected=off
  Valve_In_RL : Outport  Port=3  VectorParamsAs1DForOutWhenUnconnected=off
  Valve_In_RR : Outport  Port=4  VectorParamsAs1DForOutWhenUnconnected=off
  Valve_Out_FL : Outport  Port=5  VectorParamsAs1DForOutWhenUnconnected=off
  Valve_Out_FR : Outport  Port=6  VectorParamsAs1DForOutWhenUnconnected=off
  Valve_Out_RL : Outport  Port=7  VectorParamsAs1DForOutWhenUnconnected=off
  Valve_Out_RR : Outport  Port=8  VectorParamsAs1DForOutWhenUnconnected=off
  Valve_PV_0 : Outport  Port=9  VectorParamsAs1DForOutWhenUnconnected=off
  Valve_PV_1 : Outport  Port=10  VectorParamsAs1DForOutWhenUnconnected=off
  Valve_SV_0 : Outport  Port=11  VectorParamsAs1DForOutWhenUnconnected=off
  Valve_SV_1 : Outport  Port=12  VectorParamsAs1DForOutWhenUnconnected=off
  PumpCtrl : Outport  Port=13  VectorParamsAs1DForOutWhenUnconnected=off
  ESP_On : Outport  Port=14  VectorParamsAs1DForOutWhenUnconnected=off
  wires:
  pressure reallocation/1(Pressure deviation) -> Saturation/1
  Bus Selector/4 -> pressure reallocation/8(actual_pressure_RR)  "<Cylinder Pressure RR [bar]>"
  Bus Selector/3 -> pressure reallocation/7(actual_pressure_RL)  "<Cylinder Pressure RL [bar]>"
  Bus Selector/2 -> pressure reallocation/6(actual_pressure_FR)  "<Cylinder Pressure FR [bar]>"
  Bus Selector/1 -> pressure reallocation/5(actual_pressure_FL)  "<Cylinder Pressure FL [bar]>"
  pressure distribution target/4(brake pressure RR) -> pressure reallocation/4(target_pressure_RR)
  pressure distribution target/3(brake pressure RL) -> pressure reallocation/3(target_pressure_RL)
  pressure distribution target/2(brake pressure FR) -> pressure reallocation/2(target_pressure_FR)
  pressure distribution target/1(brake pressure FL) -> pressure reallocation/1(target_pressure_FL)
  Constant3/1 -> Product2/1
  Wheel Cylinder Pressure/1 -> Bus Selector/1
  Product1/1 -> Demux2/1
  Saturation2/1 -> Product1/1
  Product/1 -> Demux1/1
  Saturation3/1 -> Product/1
  Demux2/4 -> Valve_In_RR/1
  Demux2/3 -> Valve_In_RL/1
  Demux2/2 -> Valve_In_FR/1
  Demux2/1 -> Valve_In_FL/1
  Demux1/4 -> Valve_Out_RR/1
  Demux1/3 -> Valve_Out_RL/1
  RR_Trq_target/1 -> pressure distribution target/4(Trq Out RR)
  RL_Trq_target/1 -> pressure distribution target/3(Trq Out RL)
  Demux1/2 -> Valve_Out_FR/1
  Demux1/1 -> Valve_Out_FL/1
  Subtract2/1 -> Saturation3/1
  Subtract1/1 -> Saturation2/1
  Logical Operator2/1 -> Data Type Conversion1/1
  Logical Operator1/1 -> Logical Operator2/2, Data Type Conversion3/1
  RR_active/1 -> Logical Operator1/2
  RL_active/1 -> Logical Operator1/1
  Logical Operator/1 -> Logical Operator2/1, Data Type Conversion2/1
  FR_active/1 -> Logical Operator/2
  FL_active/1 -> Logical Operator/1
  FR_Trq_target/1 -> pressure distribution target/2(Trq Out FR)
  Constant2/1 -> Subtract2/1
  Constant1/1 -> Subtract1/1
  Saturation/1 -> Product2/2
  Product2/1 -> Subtract1/2, Subtract2/2
  FL_Trq_target/1 -> pressure distribution target/1(Trq Out FL)
  Data Type Conversion1/1 -> Product/2, Product1/2, PumpCtrl/1, ESP_On/1
  Data Type Conversion2/1 -> Valve_SV_0/1, Valve_PV_0/1
  Data Type Conversion3/1 -> Valve_SV_1/1, Valve_PV_1/1

== system ESP_RTW/ESP Controller/ESP General System/ESP/ECU ==
  ax : Inport
  Throttle Position : Inport  Port=2
  Yaw Rate : Inport  Port=3
  Steer Angle : Inport  Port=4
  Sideslip : Inport  Port=5
  mu : Inport  Port=6
  ay : Inport  Port=7
  Ideal_In : Inport  Port=8
  Vehicle Params : Inport  Port=9
  User_In : Inport  Port=10
  ECU logic : Subsystem
  Instability detectors : Subsystem
  Motor management strategy : Subsystem
  brake distribution strategy : Subsystem
  Gas_out : Outport  VectorParamsAs1DForOutWhenUnconnected=off
  FL_active : Outport  Port=2  VectorParamsAs1DForOutWhenUnconnected=off
  FL_Trq_target : Outport  Port=3  VectorParamsAs1DForOutWhenUnconnected=off
  FR_active : Outport  Port=4  VectorParamsAs1DForOutWhenUnconnected=off
  FR_Trq_target : Outport  Port=5  VectorParamsAs1DForOutWhenUnconnected=off
  RL_active : Outport  Port=6  VectorParamsAs1DForOutWhenUnconnected=off
  RL_Trq_target : Outport  Port=7  VectorParamsAs1DForOutWhenUnconnected=off
  RR_active : Outport  Port=8  VectorParamsAs1DForOutWhenUnconnected=off
  RR_Trq_target : Outport  Port=9  VectorParamsAs1DForOutWhenUnconnected=off
  wires:
  User_In/1 -> brake distribution strategy/4(User_In)
  Vehicle Params/1 -> brake distribution strategy/3(Vehicle Params), Instability detectors/7(Vehicle Params)
  Ideal_In/1 -> Instability detectors/6(Ideal_In), ECU logic/4(Ideal_In)
  mu/1 -> Instability detectors/5(mu_max), ECU logic/3(mu_max)
  Sideslip/1 -> Instability detectors/4(Sideslip)
  Instability detectors/3(motormanagement activation) -> Motor management strategy/1(activation DK)
  ay/1 -> Instability detectors/3(ay)
  Motor management strategy/1(Gas_out) -> Gas_out/1
  ax/1 -> Motor management strategy/3(ax)
  Throttle Position/1 -> Motor management strategy/2(Throttle_position)
  Instability detectors/2(YawRate corrected deviation) -> ECU logic/2(YawRate corrected deviation)
  Instability detectors/1(SideSlipAngle deviation) -> ECU logic/1(SideSlipAngle deviation)
  brake distribution strategy/8(Trq_RR_target) -> RR_Trq_target/1
  brake distribution strategy/7(RR_active) -> RR_active/1
  brake distribution strategy/6(Trq_RL_target) -> RL_Trq_target/1
  brake distribution strategy/5(RL_active) -> RL_active/1
  brake distribution strategy/4(Trq_FR_target) -> FR_Trq_target/1
  brake distribution strategy/3(FR_active) -> FR_active/1
  brake distribution strategy/2(Trq_FL_target) -> FL_Trq_target/1
  brake distribution strategy/1(FL_active) -> FL_active/1
  Yaw Rate/1 -> Instability detectors/2(Yaw Rate)
  Steer Angle/1 -> brake distribution strategy/1(Steer Angle), Instability detectors/1(Steer Angle)
  ECU logic/1(Stabilizing Torque) -> brake distribution strategy/2(Stabilizing Torque)

== system ESP_RTW/ESP Controller/ESP General System/ESP/helpsignals estimator ==
  Steer Angle : Inport
  Ideal_In : Inport  Port=2
  Vehicle Params : Inport  Port=3
  User_In : Inport  Port=4
  Bus Selector1 : BusSelector  OutputSignals=Ideal_SideSlipAngle
  Bus Selector2 : BusSelector  OutputSignals=User_estimators_on.User_SideSlip_estimator_on,User_estimators_on.User_mue_estimator_on
  Bus Selector3 : BusSelector  OutputSignals=Ideal_mu.Ideal_muFL,Ideal_mu.Ideal_muFR,Ideal_mu.Ideal_muRL,Ideal_mu.Ideal_muRR
  MinMax : MinMax  Inputs=4
  SideSlip estimator : Subsystem
  Switch : Switch  Criteria=u2 > Threshold
  Switch1 : Switch  Criteria=u2 > Threshold
  mue estimator : Subsystem
  SideslipAngle : Outport  VectorParamsAs1DForOutWhenUnconnected=off
  mu : Outport  Port=2  VectorParamsAs1DForOutWhenUnconnected=off
  wires:
  Vehicle Params/1 -> mue estimator/2(Vehicle Params)
  Bus Selector3/1 -> MinMax/1  "<Ideal_muFL>"
  Bus Selector3/4 -> MinMax/4  "<Ideal_muRR>"
  Bus Selector3/2 -> MinMax/2  "<Ideal_muFR>"
  Bus Selector3/3 -> MinMax/3  "<Ideal_muRL>"
  Ideal_In/1 -> Bus Selector1/1, SideSlip estimator/2(CarMaker_In), mue estimator/1(CarMaker_In), Bus Selector3/1
  MinMax/1 -> Switch1/3
  Switch1/1 -> mu/1
  Bus Selector2/2 -> Switch1/2  "<User_mue_estimator_on>"
  Switch/1 -> SideslipAngle/1
  SideSlip estimator/1(SideSlipAngle_estimated) -> Switch/1
  Bus Selector1/1 -> Switch/3  "<Ideal_SideSlipAngle>"
  Bus Selector2/1 -> Switch/2  "<User_SideSlip_estimator_on>"
  User_In/1 -> Bus Selector2/1
  mue estimator/1(mue_estimated) -> Switch1/1
  Steer Angle/1 -> SideSlip estimator/1(lenkwinkel)

== system ESP_RTW/ESP Controller/ESP General System/Master Controller/ABS Off ==
  ABS On : Inport
  ABS Bus : Inport  Port=2
  Bus Creator : BusCreator  Inputs=8
  Bus Creator4 : BusCreator  Inputs='Pilot Valves','Suction Valves','Brake Valves','Pump Ctrl'
  Bus Selector1 : BusSelector  OutputSignals=Valve_In_FL,Valve_In_FR,Valve_In_RL,Valve_In_RR,Valve_Out_FL,Valve_Out_FR,Valve_Out_RL,Valve_Out_RR
  Bus Selector3 : BusSelector  OutputSignals=Pilot Valves,Suction Valves,Brake Valves,Pump Ctrl
  Product{,1..7} (8 alike) : Product  RndMeth=Zero
  ABS Bus Out : Outport  VectorParamsAs1DForOutWhenUnconnected=off
  wires:
  Product7/1 -> Bus Creator/8  "Valve_Out_RR"
  Bus Selector1/8 -> Product7/2  "<Valve_Out_RR>"
  Product6/1 -> Bus Creator/7  "Valve_Out_RL"
  Bus Selector1/7 -> Product6/2  "<Valve_Out_RL>"
  Product5/1 -> Bus Creator/6  "Valve_Out_FR"
  Bus Selector1/6 -> Product5/2  "<Valve_Out_FR>"
  Product4/1 -> Bus Creator/5  "Valve_Out_FL"
  Bus Selector1/5 -> Product4/2  "<Valve_Out_FL>"
  Product3/1 -> Bus Creator/4  "Valve_In_RR"
  Bus Selector1/4 -> Product3/2  "<Valve_In_RR>"
  Product2/1 -> Bus Creator/3  "Valve_In_RL"
  Bus Selector1/3 -> Product2/2  "<Valve_In_RL>"
  Product1/1 -> Bus Creator/2  "Valve_In_FR"
  Bus Selector1/2 -> Product1/2  "<Valve_In_FR>"
  Product/1 -> Bus Creator/1  "Valve_In_FL"
  Bus Selector1/1 -> Product/2  "<Valve_In_FL>"
  ABS On/1 -> Product/1, Product1/1, Product2/1, Product3/1, Product4/1, Product5/1, Product6/1, Product7/1
  Bus Creator/1 -> Bus Creator4/3  "Brake Valves"
  Bus Selector3/4 -> Bus Creator4/4  "<Pump Ctrl>"
  Bus Selector3/3 -> Bus Selector1/1  "<Brake Valves>"
  Bus Selector3/2 -> Bus Creator4/2  "<Suction Valves>"
  Bus Selector3/1 -> Bus Creator4/1  "<Pilot Valves>"
  ABS Bus/1 -> Bus Selector3/1
  Bus Creator4/1 -> ABS Bus Out/1  "ABS Bus"

== system ESP_RTW/ESP Controller/ESP General System/Master Controller/Actuator VC ==
  VC_IN : Inport
  HSA_BrakePark : Inport  Port=2
  Gas_Out_ASR : Inport  Port=3
  Gas_Out_ESP : Inport  Port=4
  HSA_Flag : Inport  Port=5
  ASR_Flag : Inport  Port=6
  ESP_Flag : Inport  Port=7
  Bus Selector3 : BusSelector  OutputSignals=Gas,Park
  Bus Creator : BusCreator  Inputs=2
  Constant : Constant
  MinMax : MinMax  Inputs=3
  MinMax1 : MinMax  Function=max  Inputs=2
  Product : Product  RndMeth=Zero
  Subtract1 : Sum  Inputs=+-+
  Subtract2 : Sum  Inputs=+-+
  VC_OUT : Outport  VectorParamsAs1DForOutWhenUnconnected=off
  wires:
  ESP_Flag/1 -> Subtract2/2
  MinMax/1 -> Bus Creator/1  "VC_Gas"
  Bus Creator/1 -> VC_OUT/1
  MinMax1/1 -> Bus Creator/2  "VC_BrakePark"
  Product/1 -> MinMax1/2
  HSA_BrakePark/1 -> Product/2
  HSA_Flag/1 -> Product/1
  Bus Selector3/2 -> MinMax1/1  "<Park>"
  Bus Selector3/1 -> MinMax/3  "<Gas>"
  VC_IN/1 -> Bus Selector3/1
  Subtract1/1 -> MinMax/2
  Gas_Out_ASR/1 -> Subtract1/3
  ASR_Flag/1 -> Subtract1/2
  Subtract2/1 -> MinMax/1
  Gas_Out_ESP/1 -> Subtract2/3
  Constant/1 -> Subtract2/1, Subtract1/1

== system ESP_RTW/ESP Controller/ESP General System/Master Controller/User Switch ==
  ESP On : Inport
  ASR On : Inport  Port=2
  ABS On : Inport  Port=3
  HSA On : Inport  Port=4
  User In : Inport  Port=5
  Bus Creator6 : BusCreator  Inputs=3
  Bus Selector : BusSelector  OutputSignals=ASR On,MSR On,BMR On
  Bus Selector4 : BusSelector  OutputSignals=User_Switch.User_Switch_Main_off,User_Switch.User_Switch_ESP_off,User_Switch.User_Switch_ASR_off,User_Switch.User_Switch_ABS_off,User_Switch.User_Switch_HSA_off
  Constant : Constant
  Product{,1..9} (10 alike) : Product  RndMeth=Zero
  Subtract{,1..4} (5 alike) : Sum  Inputs=+-
  "ESP On " : Outport  VectorParamsAs1DForOutWhenUnconnected=off
  "ASR On " : Outport  Port=2  VectorParamsAs1DForOutWhenUnconnected=off
  "ABS On " : Outport  Port=3  VectorParamsAs1DForOutWhenUnconnected=off
  "HSA On " : Outport  Port=4  VectorParamsAs1DForOutWhenUnconnected=off
  ASRASR On : Outport  Port=5  VectorParamsAs1DForOutWhenUnconnected=off
  wires:
  Product9/1 -> "HSA On "/1  "HSA On"
  HSA On/1 -> Product9/2
  Product8/1 -> Product9/1
  Subtract4/1 -> Product8/2
  Bus Selector4/5 -> Subtract4/2  "<User_Switch_HSA_off>"
  User In/1 -> Bus Selector4/1
  Product7/1 -> "ABS On "/1  "ABS On"
  ABS On/1 -> Product7/2
  Product2/1 -> Product7/1
  Product6/1 -> Bus Creator6/3  "BMR On"
  Bus Selector/3 -> Product6/2  "<BMR On>"
  Bus Creator6/1 -> "ASR On "/1  "ASR On"
  Product5/1 -> Bus Creator6/2  "MSR On"
  Bus Selector/2 -> Product5/2  "<MSR On>"
  Product4/1 -> ASRASR On/1, Bus Creator6/1  "ASR On"
  Bus Selector/1 -> Product4/2  "<ASR On>"
  Product1/1 -> Product4/1, Product5/1, Product6/1
  Product3/1 -> "ESP On "/1  "ESP On"
  ESP On/1 -> Product3/2
  Product/1 -> Product3/1
  Subtract3/1 -> Product2/2
  Subtract2/1 -> Product1/2
  Subtract1/1 -> Product/2
  Subtract/1 -> Product2/1, Product8/1, Product1/1, Product/1
  Bus Selector4/4 -> Subtract3/2  "<User_Switch_ABS_off>"
  Bus Selector4/3 -> Subtract2/2  "<User_Switch_ASR_off>"
  Bus Selector4/2 -> Subtract1/2  "<User_Switch_ESP_off>"
  Bus Selector4/1 -> Subtract/2  "<User_Switch_Main_off>"
  Constant/1 -> Subtract/1, Subtract1/1, Subtract2/1, Subtract3/1, Subtract4/1
  ASR On/1 -> Bus Selector/1

== system ESP_RTW/ESP Controller/ESP General System/ABS/ABS ECU/ABS_ValveCtrl_FL ==
  note: EITHER ABS is switched on and  S_K is put through
      |  when S_K is becomming bigger the s_{ku}
      | OR output is 0 when S_K is smaller than {sku}_{off}
  note: Valve Control:
      | Valves are open for a predefined time window.
      | The driving time depends on a trigger criterion (LUT).
      | The treshold change for the valve driving time is
      | continously modified by a repeating sequence.
  note: Control strategy: Trigger criterion S_K
      | S_K combines wheel decceleration control with slip control
      | using weighting factors  K_z and K_\lambda
      | S_K=K_z*z_R + K_\lambda * \lambda_{rel}
      | (see p.127 in M. Burckhardt
      | Fahrwerktechnik:Radschlupfregelsysteme)
  slip : Inport
  wheelspeed : Inport  Port=2
  rstat : Inport  Port=3
  Constant : Constant
  Constant1 : Constant  Value=f_slip
  Constant3 : Constant  Value=f_ax
  Derivative : Derivative
  Duty : Subsystem
  Look-Up Table1 : Lookup  InputValues=Valve_LUTin_VA  Table=ValveIn_LUTout_VA  LookUpMeth=Interpolation-Use End Values  SaturateOnIntegerOverflow=on
  Look-Up Table2 : Lookup  InputValues=Valve_LUTin_VA  Table=ValveOut_LUTout_VA  LookUpMeth=Interpolation-Use End Values  SaturateOnIntegerOverflow=on
  Product : Product  SaturateOnIntegerOverflow=on  OutDataTypeStr=Inherit: Same as first input
  Product1 : Product  Inputs=3  InputSameDT=on  SaturateOnIntegerOverflow=on  OutDataTypeStr=Inherit: Same as first input
  Product2 : Product  SaturateOnIntegerOverflow=on  OutDataTypeStr=Inherit: Same as first input
  Rate Transition{1..4} (4 alike) : RateTransition
  Relational Operator : RelationalOperator  Operator=<  SampleTime=0.001  RndMeth=Nearest
  Relational Operator1 : RelationalOperator  Operator=<  SampleTime=0.001  RndMeth=Nearest
  Relay : Relay  OnSwitchValue=sku_VA  OffSwitchValue=sku_off_VA
  Sum : Sum  Inputs=|--  InputSameDT=on  SaturateOnIntegerOverflow=on  OutDataTypeStr=Inherit: Same as first input
  Sum1 : Sum  Inputs=--+  SaturateOnIntegerOverflow=on
  Zero-Order Hold : ZeroOrderHold  SampleTime=t_Sensor
  Brake.Valve.In : Outport  VectorParamsAs1DForOutWhenUnconnected=off
  Brake.Valve.Out : Outport  Port=2  VectorParamsAs1DForOutWhenUnconnected=off
  Brake.ABS.status : Outport  Port=3  VectorParamsAs1DForOutWhenUnconnected=off
  Brake.ABS.on/off : Outport  Port=4  VectorParamsAs1DForOutWhenUnconnected=off
  wires:
  Rate Transition2/1 -> Relational Operator1/1, Relational Operator/1
  Rate Transition4/1 -> Brake.ABS.on/off/1
  Rate Transition3/1 -> Relational Operator1/2
  Rate Transition1/1 -> Relational Operator/2
  Duty/1(SZ) -> Rate Transition2/1
  Constant1/1 -> Product2/1
  Derivative/1 -> Product1/1
  Product2/1 -> Sum/1
  Product1/1 -> Sum/2
  slip/1 -> Product2/2
  wheelspeed/1 -> Derivative/1
  rstat/1 -> Product1/2
  Constant3/1 -> Product1/3
  Relational Operator/1 -> Brake.Valve.In/1, Sum1/1
  Relational Operator1/1 -> Sum1/2, Brake.Valve.Out/1
  Constant/1 -> Sum1/3
  Sum1/1 -> Brake.ABS.status/1
  Sum/1 -> Zero-Order Hold/1  "S_K"
  Product/1 -> Look-Up Table2/1, Look-Up Table1/1
  Look-Up Table1/1 -> Rate Transition1/1
  Look-Up Table2/1 -> Rate Transition3/1
  Relay/1 -> Product/2, Rate Transition4/1
  Zero-Order Hold/1 -> Relay/1, Product/1

== system ESP_RTW/ESP Controller/ESP General System/ABS/ABS ECU/ABS_ValveCtrl_FR ==
  note: EITHER ABS is switched on and  S_K is put through
      |  when S_K is becomming bigger the s_{ku}
      | OR output is 0 when S_K is smaller than {sku}_{off}
  note: Valve Control:
      | Valves are open for a predefined time window.
      | The driving time depends on a trigger criterion (LUT).
      | The treshold change for the valve driving time is
      | continously modified by a repeating sequence.
  note: Control strategy: Trigger criterion S_K
      | S_K combines wheel decceleration control with slip control
      | using weighting factors  K_z and K_\lambda
      | S_K=K_z*z_R + K_\lambda * \lambda_{rel}
      | (see p.127 in M. Burckhardt
      | Fahrwerktechnik:Radschlupfregelsysteme)
  slip : Inport
  wheelspeed : Inport  Port=2
  rstat : Inport  Port=3
  Constant : Constant
  Constant1 : Constant  Value=f_slip
  Constant3 : Constant  Value=f_ax
  Derivative : Derivative
  Duty : Subsystem
  Look-Up Table1 : Lookup  InputValues=Valve_LUTin_VA  Table=ValveIn_LUTout_VA  LookUpMeth=Interpolation-Use End Values  SaturateOnIntegerOverflow=on
  Look-Up Table2 : Lookup  InputValues=Valve_LUTin_VA  Table=ValveOut_LUTout_VA  LookUpMeth=Interpolation-Use End Values  SaturateOnIntegerOverflow=on
  Product : Product  SaturateOnIntegerOverflow=on  OutDataTypeStr=Inherit: Same as first input
  Product1 : Product  Inputs=3  InputSameDT=on  SaturateOnIntegerOverflow=on  OutDataTypeStr=Inherit: Same as first input
  Product2 : Product  SaturateOnIntegerOverflow=on  OutDataTypeStr=Inherit: Same as first input
  Rate Transition{1..4} (4 alike) : RateTransition
  Relational Operator : RelationalOperator  Operator=<  SampleTime=0.001  RndMeth=Nearest
  Relational Operator1 : RelationalOperator  Operator=<  SampleTime=0.001  RndMeth=Nearest
  Relay : Relay  OnSwitchValue=sku_VA  OffSwitchValue=sku_off_VA
  Sum : Sum  Inputs=|--  InputSameDT=on  SaturateOnIntegerOverflow=on  OutDataTypeStr=Inherit: Same as first input
  Sum1 : Sum  Inputs=--+  SaturateOnIntegerOverflow=on
  Zero-Order Hold : ZeroOrderHold  SampleTime=t_Sensor
  Brake.Valve.In : Outport  VectorParamsAs1DForOutWhenUnconnected=off
  Brake.Valve.Out : Outport  Port=2  VectorParamsAs1DForOutWhenUnconnected=off
  Brake.ABS.status : Outport  Port=3  VectorParamsAs1DForOutWhenUnconnected=off
  Brake.ABS.on/off : Outport  Port=4  VectorParamsAs1DForOutWhenUnconnected=off
  wires:
  Rate Transition4/1 -> Brake.ABS.on/off/1
  Rate Transition3/1 -> Relational Operator1/2
  Rate Transition1/1 -> Relational Operator/2
  Rate Transition2/1 -> Relational Operator1/1, Relational Operator/1
  Constant1/1 -> Product2/1
  Derivative/1 -> Product1/1
  Product2/1 -> Sum/1
  Product1/1 -> Sum/2
  slip/1 -> Product2/2
  wheelspeed/1 -> Derivative/1
  rstat/1 -> Product1/2
  Constant3/1 -> Product1/3
  Relational Operator/1 -> Brake.Valve.In/1, Sum1/1
  Relational Operator1/1 -> Brake.Valve.Out/1, Sum1/2
  Constant/1 -> Sum1/3
  Sum1/1 -> Brake.ABS.status/1
  Sum/1 -> Zero-Order Hold/1
  Product/1 -> Look-Up Table1/1, Look-Up Table2/1
  Duty/1(SZ) -> Rate Transition2/1
  Look-Up Table1/1 -> Rate Transition1/1
  Look-Up Table2/1 -> Rate Transition3/1
  Relay/1 -> Product/2, Rate Transition4/1
  Zero-Order Hold/1 -> Relay/1, Product/1
